simulink model "AFE_art"  (R2019b)
settings: Solver=FixedStepAuto  StartTime=0.0  StopTime=10.0  FixedStep=fixedStepSize  RelTol=1e-3
undefined symbols (not defined in the file): artificial_AFE_RFC_max, artificial_AFE_RFC_min, artificial_AFE_time, artificial_AOT_AFE_max, artificial_AOT_AFE_min
settings Model: Creator=JEDDELAN  LastModifiedBy=jeddelan
settings DataIOCC: SaveOutput=off  SaveTime=off  ReturnWorkspaceOutputs=off
settings DebuggingCC: ArithmeticOperatorsInVariantConditions=warning
settings SFSimCC: SimUseLocalCustomCode=off  CustomCodeUndefinedFunction=UseInterfaceOnly
settings RTWCC: RTWUseLocalCustomCode=off
settings GRTTargetCC: CombineOutputUpdateFcns=off  MatFileLogging=off

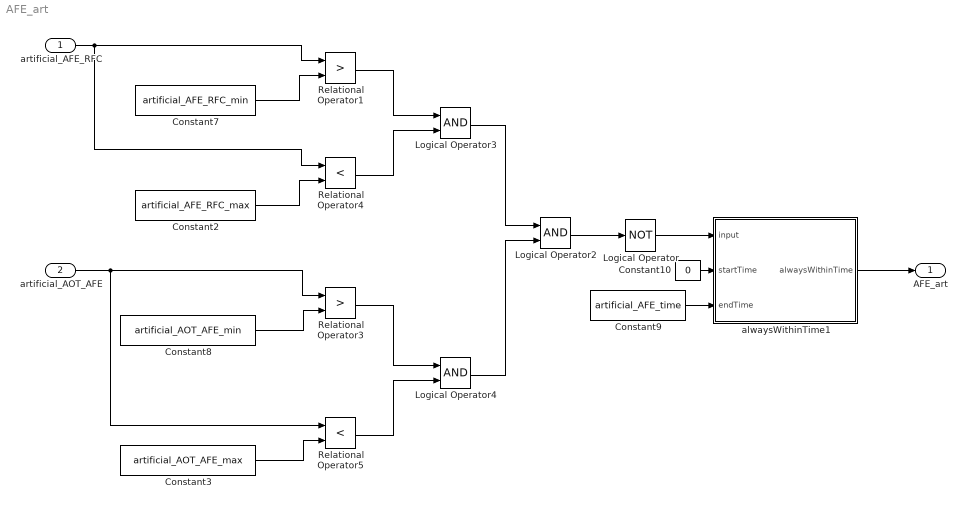
== system AFE_art ==
  artificial_AFE_RFC : Inport
  artificial_AOT_AFE : Inport  Port=2
  Constant10 : Constant  Value=0
  Constant2 : Constant  Value=artificial_AFE_RFC_max
  Constant3 : Constant  Value=artificial_AOT_AFE_max
  Constant7 : Constant  Value=artificial_AFE_RFC_min
  Constant8 : Constant  Value=artificial_AOT_AFE_min
  Constant9 : Constant  Value=artificial_AFE_time
  Logical Operator : Logic  Operator=NOT  AllPortsSameDT=off  OutDataTypeStr=boolean
  Logical Operator2 : Logic  AllPortsSameDT=off  OutDataTypeStr=boolean
  Logical Operator3 : Logic  AllPortsSameDT=off  OutDataTypeStr=boolean
  Logical Operator4 : Logic  AllPortsSameDT=off  OutDataTypeStr=boolean
  Relational Operator1 : RelationalOperator  Operator=>  OutDataTypeStr=boolean  RndMeth=Simplest
  Relational Operator3 : RelationalOperator  Operator=>  OutDataTypeStr=boolean  RndMeth=Simplest
  Relational Operator4 : RelationalOperator  Operator=<  OutDataTypeStr=boolean  RndMeth=Simplest
  Relational Operator5 : RelationalOperator  Operator=<  OutDataTypeStr=boolean  RndMeth=Simplest
  alwaysWithinTime1 : Subsystem
      settings: CopyFcn=set_param(gcbh,'LinkStatus','none');
  AFE_art : Outport  OutDataTypeStr=boolean  PortDimensions=1  VectorParamsAs1DForOutWhenUnconnected=off
  wires:
  artificial_AFE_RFC/1 -> Relational Operator4/1, Relational Operator1/1
  Relational Operator1/1 -> Logical Operator3/1
  Relational Operator4/1 -> Logical Operator3/2
  Constant3/1 -> Relational Operator5/2
  Relational Operator3/1 -> Logical Operator4/1
  Logical Operator3/1 -> Logical Operator2/1
  Constant8/1 -> Relational Operator3/2
  alwaysWithinTime1/1(alwaysWithinTime) -> AFE_art/1
  Constant9/1 -> alwaysWithinTime1/3(endTime)
  Constant2/1 -> Relational Operator4/2
  Logical Operator4/1 -> Logical Operator2/2
  Constant10/1 -> alwaysWithinTime1/2(startTime)
  Logical Operator/1 -> alwaysWithinTime1/1(input)
  artificial_AOT_AFE/1 -> Relational Operator5/1, Relational Operator3/1
  Logical Operator2/1 -> Logical Operator/1
  Relational Operator5/1 -> Logical Operator4/2
  Constant7/1 -> Relational Operator1/2

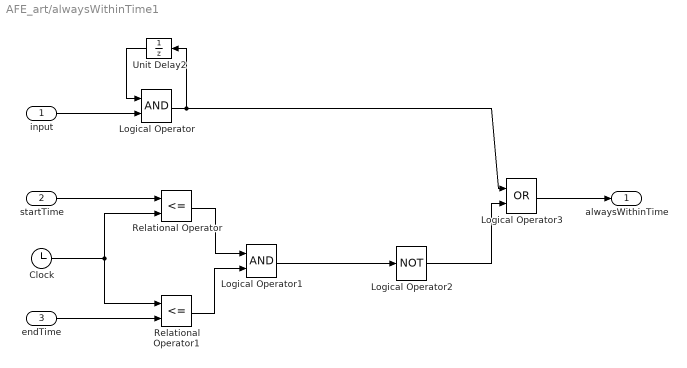
== system AFE_art/alwaysWithinTime1 ==
  input : Inport
  startTime : Inport  Port=2
  endTime : Inport  Port=3
  Clock : Clock
  Logical Operator : Logic  AllPortsSameDT=off  OutDataTypeStr=boolean
  Logical Operator1 : Logic  AllPortsSameDT=off  OutDataTypeStr=boolean
  Logical Operator2 : Logic  Operator=NOT  AllPortsSameDT=off  OutDataTypeStr=boolean
  Logical Operator3 : Logic  Operator=OR  AllPortsSameDT=off  OutDataTypeStr=boolean
  Relational Operator : RelationalOperator  Operator=<=  OutDataTypeStr=boolean  RndMeth=Simplest
  Relational Operator1 : RelationalOperator  Operator=<=  OutDataTypeStr=boolean  RndMeth=Simplest
  Unit Delay2 : UnitDelay  InitialCondition=1  SampleTime=-1  HasFrameUpgradeWarning=on
  alwaysWithinTime : Outport  VectorParamsAs1DForOutWhenUnconnected=off
  wires:
  startTime/1 -> Relational Operator/1
  Unit Delay2/1 -> Logical Operator/1
  input/1 -> Logical Operator/2
  Logical Operator/1 -> Logical Operator3/1, Unit Delay2/1
  Clock/1 -> Relational Operator1/1, Relational Operator/2
  endTime/1 -> Relational Operator1/2
  Relational Operator1/1 -> Logical Operator1/2
  Relational Operator/1 -> Logical Operator1/1
  Logical Operator1/1 -> Logical Operator2/1
  Logical Operator2/1 -> Logical Operator3/2
  Logical Operator3/1 -> alwaysWithinTime/1
